simulink model "MODELO"  (R2024a)
settings: Solver=VariableStepAuto  StartTime=0.0  StopTime=10  RelTol=1e-3
libraries: simulink x2
settings Model: Creator=LENOVO  LastModifiedBy=LENOVO

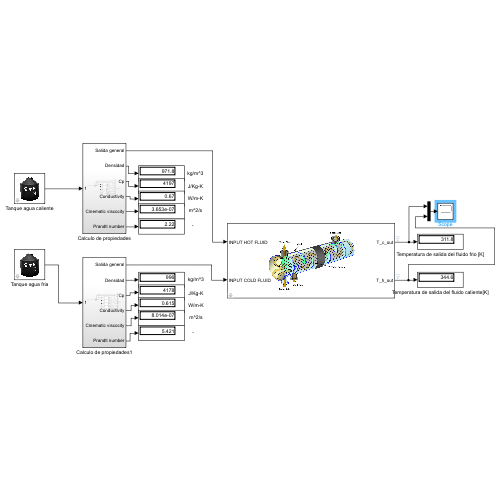
[thumbnail: Simulink's stored preview of the top-level diagram]
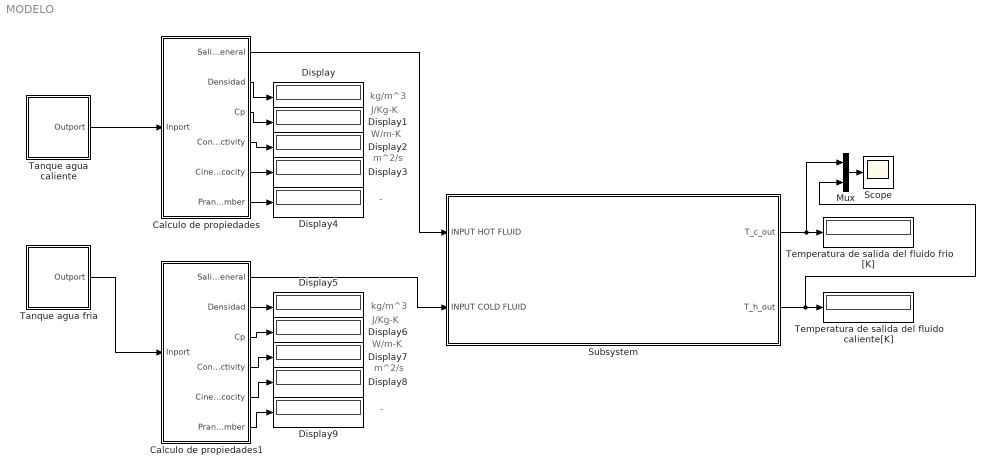
== system MODELO ==
  note: -
  note: m^2/s
  note: W/m-K
  note: J/Kg-K
  note: kg/m^3
  note: W/m-K
  note: -
  note: kg/m^3
  note: m^2/s
  note: J/Kg-K
  Calculo de propiedades : Subsystem
  Calculo de propiedades1 : Subsystem
  Display{,1..9} (10 alike) : Display
  Mux : Mux  Inputs=2
  Scope : Scope
  Subsystem : Subsystem  mask{jc=1.05, jl=1, jb=1, js=0.7065, jr=1, rfi=0, rfo=0}
      mask prompts: rfi "Factor de ensuciemiento dentro de los tubos"; rfo "Factor de ensuciemiento de la coraza"
      mask DialogControl Control2 Prompt: Introduzca los factores de corrección dados por el método de Bell-Delaware
      mask DialogControl Control3 Prompt: Introduzca los factores de ensuciamiento
      mask Display: image('HX.png', [0,0,0,0,90,90]);
  Tanque agua caliente : Subsystem  mask{Temp=80+273.15, ifCaudal=off, caudal=90, m_dot=10, area=2}
      mask prompts: Temp "Temperatura"; ifCaudal "Usar caudal"; m_dot "Flujo másico"
      mask Display: image('tanque_img.webp');
  Tanque agua fria : Subsystem  mask{Temp=30+273.15, ifCaudal=off, caudal=90, m_dot=3, area=2}
      mask prompts: Temp "Temperatura"; ifCaudal "Usar caudal"; m_dot "Flujo másico"
      mask Display: image('tanque_img.webp');
  Temperatura de salida del fluido caliente[K] : Display
  Temperatura de salida del fluido frio [K] : Display
  wires:
  Tanque agua caliente/1(Outport) -> Calculo de propiedades/1(Inport)
  Calculo de propiedades/2(Densidad) -> Display/1
  Calculo de propiedades/3(Cp) -> Display1/1
  Calculo de propiedades/4(Conductivity) -> Display2/1
  Calculo de propiedades/5(Cinematic viscocity) -> Display3/1
  Calculo de propiedades/6(Prandtl number) -> Display4/1
  Calculo de propiedades/1(Salida general) -> Subsystem/1(INPUT HOT FLUID)
  Tanque agua fria/1(Outport) -> Calculo de propiedades1/1(Inport)
  Calculo de propiedades1/2(Densidad) -> Display5/1
  Calculo de propiedades1/3(Cp) -> Display6/1
  Calculo de propiedades1/4(Conductivity) -> Display7/1
  Calculo de propiedades1/5(Cinematic viscocity) -> Display8/1
  Calculo de propiedades1/6(Prandtl number) -> Display9/1
  Calculo de propiedades1/1(Salida general) -> Subsystem/2(INPUT COLD FLUID)
  Subsystem/1(T_c_out) -> Mux/1, Temperatura de salida del fluido frio [K]/1
  Subsystem/2(T_h_out) -> Mux/2, Temperatura de salida del fluido caliente[K]/1
  Mux/1 -> Scope/1

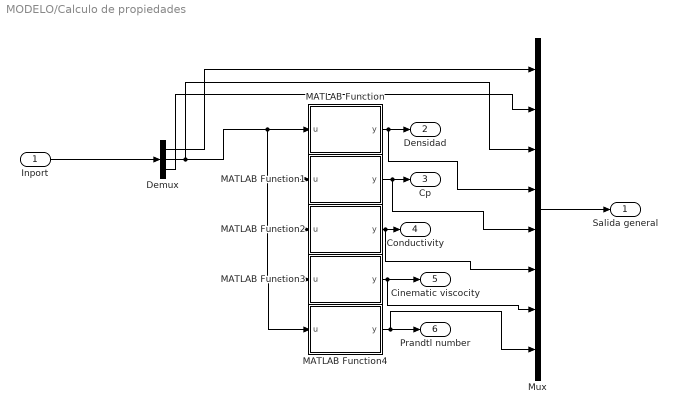
== system MODELO/Calculo de propiedades ==
  Inport : Inport
  Demux : Demux  Outputs=3
  MATLAB Function : MATLAB Function  TreatAsAtomicUnit=on
  MATLAB Function1 : MATLAB Function  TreatAsAtomicUnit=on
  MATLAB Function2 : MATLAB Function  TreatAsAtomicUnit=on
  MATLAB Function3 : MATLAB Function  TreatAsAtomicUnit=on
  MATLAB Function4 : MATLAB Function  TreatAsAtomicUnit=on
  Mux : Mux  Inputs=8
  Salida general : Outport
  Densidad : Outport  Port=2
  Cp : Outport  Port=3
  Conductivity : Outport  Port=4
  Cinematic viscocity : Outport  Port=5
  Prandtl number : Outport  Port=6
  wires:
  Inport/1 -> Demux/1
  Demux/1 -> Mux/1
  Demux/2 -> Mux/3, MATLAB Function4/1(u), MATLAB Function3/1(u), MATLAB Function2/1(u), MATLAB Function1/1(u), MATLAB Function/1(u)
  Demux/3 -> Mux/2
  MATLAB Function/1(y) -> Mux/4, Densidad/1
  MATLAB Function1/1(y) -> Mux/5, Cp/1
  MATLAB Function2/1(y) -> Mux/6, Conductivity/1
  MATLAB Function3/1(y) -> Mux/7, Cinematic viscocity/1
  MATLAB Function4/1(y) -> Mux/8, Prandtl number/1
  Mux/1 -> Salida general/1

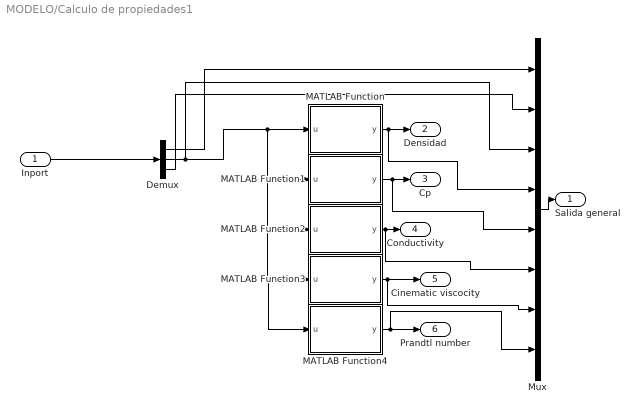
== system MODELO/Calculo de propiedades1 ==
  Inport : Inport
  Demux : Demux  Outputs=3
  MATLAB Function : MATLAB Function  TreatAsAtomicUnit=on
  MATLAB Function1 : MATLAB Function  TreatAsAtomicUnit=on
  MATLAB Function2 : MATLAB Function  TreatAsAtomicUnit=on
  MATLAB Function3 : MATLAB Function  TreatAsAtomicUnit=on
  MATLAB Function4 : MATLAB Function  TreatAsAtomicUnit=on
  Mux : Mux  Inputs=8
  Salida general : Outport
  Densidad : Outport  Port=2
  Cp : Outport  Port=3
  Conductivity : Outport  Port=4
  Cinematic viscocity : Outport  Port=5
  Prandtl number : Outport  Port=6
  wires:
  Inport/1 -> Demux/1
  Demux/1 -> Mux/1
  Demux/2 -> Mux/3, MATLAB Function4/1(u), MATLAB Function3/1(u), MATLAB Function2/1(u), MATLAB Function1/1(u), MATLAB Function/1(u)
  Demux/3 -> Mux/2
  MATLAB Function/1(y) -> Mux/4, Densidad/1
  MATLAB Function1/1(y) -> Mux/5, Cp/1
  MATLAB Function2/1(y) -> Mux/6, Conductivity/1
  MATLAB Function3/1(y) -> Mux/7, Cinematic viscocity/1
  MATLAB Function4/1(y) -> Mux/8, Prandtl number/1
  Mux/1 -> Salida general/1

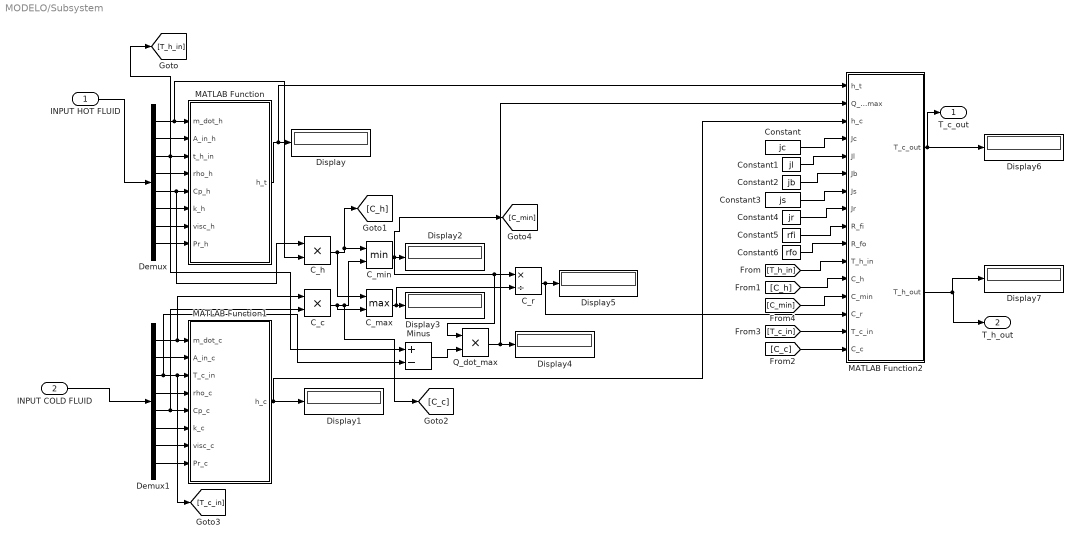
== system MODELO/Subsystem ==
  INPUT HOT FLUID : Inport
  INPUT COLD FLUID : Inport  Port=2
  C_c : Product
  C_h : Product
  C_max : MinMax  Function=max  Inputs=2
  C_min : MinMax  Inputs=2
  C_r : Product  Inputs=*/
  Constant : Constant  Value=jc
  Constant1 : Constant  Value=jl
  Constant2 : Constant  Value=jb
  Constant3 : Constant  Value=js
  Constant4 : Constant  Value=jr
  Constant5 : Constant  Value=rfi
  Constant6 : Constant  Value=rfo
  Demux : Demux  Outputs=8
  Demux1 : Demux  Outputs=8
  Display{,1..7} (8 alike) : Display
  MATLAB Function : MATLAB Function  TreatAsAtomicUnit=on
  MATLAB Function1 : MATLAB Function  TreatAsAtomicUnit=on
  MATLAB Function2 : MATLAB Function  TreatAsAtomicUnit=on
  Minus : Sum  Inputs=+-
  Q_dot_max : Product
  T_c_out : Outport
  T_h_out : Outport  Port=2
  wires:
  INPUT HOT FLUID/1 -> Demux/1
  Demux/1 -> C_h/2, MATLAB Function/1(m_dot_h)
  Demux/2 -> MATLAB Function/2(A_in_h)
  Demux/3 -> [T_h_in], Minus/1, MATLAB Function/3(t_h_in)
  Demux/4 -> MATLAB Function/4(rho_h)
  Demux/7 -> MATLAB Function/7(visc_h)
  Demux/8 -> MATLAB Function/8(Pr_h)
  Demux1/1 -> C_c/1, MATLAB Function1/1(m_dot_c)
  Demux1/2 -> MATLAB Function1/2(A_in_c)
  Demux1/3 -> Minus/2, [T_c_in], MATLAB Function1/3(T_c_in)
  Demux1/4 -> MATLAB Function1/4(rho_c)
  Demux1/5 -> C_c/2, MATLAB Function1/5(Cp_c)
  Demux1/6 -> MATLAB Function1/6(k_c)
  Demux1/7 -> MATLAB Function1/7(visc_c)
  Demux1/8 -> MATLAB Function1/8(Pr_c)
  INPUT COLD FLUID/1 -> Demux1/1
  MATLAB Function/1(h_t) -> MATLAB Function2/1(h_t), Display/1
  MATLAB Function1/1(h_c) -> MATLAB Function2/3(h_c), Display1/1
  Demux/5 -> C_h/1, MATLAB Function/5(Cp_h)
  Demux/6 -> MATLAB Function/6(k_h)
  C_h/1 -> C_max/1, [C_h], C_min/1
  C_c/1 -> C_max/2, [C_c], C_min/2
  C_max/1 -> C_r/2, Display3/1
  C_min/1 -> [C_min], Q_dot_max/1, C_r/1, Display2/1
  Minus/1 -> Q_dot_max/2
  Q_dot_max/1 -> MATLAB Function2/2(Q_dot_max), Display4/1
  C_r/1 -> MATLAB Function2/14(C_r), Display5/1
  Constant/1 -> MATLAB Function2/4(Jc)
  Constant2/1 -> MATLAB Function2/6(Jb)
  Constant1/1 -> MATLAB Function2/5(Jl)
  Constant3/1 -> MATLAB Function2/7(Js)
  Constant4/1 -> MATLAB Function2/8(Jr)
  Constant5/1 -> MATLAB Function2/9(R_fi)
  Constant6/1 -> MATLAB Function2/10(R_fo)
  [T_h_in] -> MATLAB Function2/11(T_h_in)
  [C_h] -> MATLAB Function2/12(C_h)
  [C_c] -> MATLAB Function2/16(C_c)
  [T_c_in] -> MATLAB Function2/15(T_c_in)
  [C_min] -> MATLAB Function2/13(C_min)
  MATLAB Function2/1(T_c_out) -> T_c_out/1, Display6/1
  MATLAB Function2/2(T_h_out) -> Display7/1, T_h_out/1

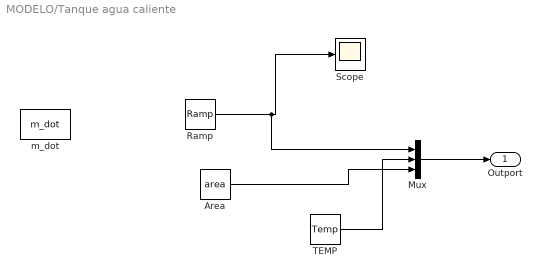
== system MODELO/Tanque agua caliente ==
  Area : Constant  Value=area
  Mux : Mux  Inputs=3
  Ramp : simulink/Sources/Ramp  slope=1  start=0  InitialOutput=0
  Scope : Scope
  TEMP : Constant  Value=Temp
  m_dot : Constant  Value=m_dot
  Outport : Outport
  wires:
  TEMP/1 -> Mux/2
  Area/1 -> Mux/3
  Mux/1 -> Outport/1
  Ramp/1 -> Mux/1, Scope/1

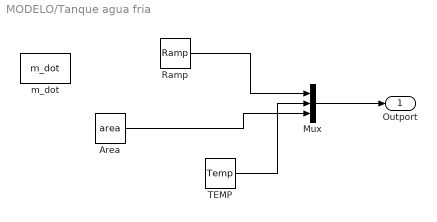
== system MODELO/Tanque agua fria ==
  Area : Constant  Value=area
  Mux : Mux  Inputs=3
  Ramp : simulink/Sources/Ramp  slope=1  start=0  InitialOutput=0
  TEMP : Constant  Value=Temp
  m_dot : Constant  Value=m_dot
  Outport : Outport
  wires:
  TEMP/1 -> Mux/2
  Area/1 -> Mux/3
  Mux/1 -> Outport/1
  Ramp/1 -> Mux/1

== matlab function MODELO/Calculo de propiedades1/MATLAB Function2 ==
  data: u input; y output
function y = fcn(u)
    temp_vector=273.16:5:373.16;
    k_vector = [0.56 0.571 0.580 0.589 0.598 0.607 0.615 0.623 0.631 0.637 ...
            0.644 0.649 0.654 0.659 0.663 0.667 0.670 0.673 0.675 0.677 ...
            0.679];
    fluid_k = interp1(temp_vector, k_vector, u);

y = fluid_k;

== matlab function MODELO/Calculo de propiedades1/MATLAB Function3 ==
  data: u input; y output
function y = fcn(u)
    temp_vector=273.16:5:373.16;
    density_vector=[999.8 999.9 999.7 999.1 998.0 997.0 996.0 994.0 992.1 990.1 988.1 985.2 983.3 980.4 977.5 974.7 971.8 968.1 965.3 961.5 957.9];
    mu_vector = [1.792e-3 1.519e-3 1.307e-3 1.138e-3 1.002e-3 ...
             0.891e-3 0.798e-3 0.720e-3 0.653e-3 0.596e-3 ...
             0.547e-3 0.467e-3 0.467e-3 0.433e-3 0.404e-3 ...
             0.378e-3 0.355e-3 0.333e-3 0.315e-3 0.297e-3 ...
             0.282e-3];
    v_vector=mu_vector./density_vector;
    
    fluid_v = interp1(temp_vector, v_vector, u);

y = fluid_v;

== matlab function MODELO/Calculo de propiedades1/MATLAB Function4 ==
  data: u input; y output
function y = fcn(u)
    temp_vector=273.16:5:373.16;
    pr_vector = [13.5 11.2 9.45 8.09 7.01 6.14 5.42 4.83 ...
             4.32 3.91 3.55 3.25 2.99 2.75 2.55 2.38 ...
             2.22 2.08 1.96 1.85 1.75];
    fluid_pr = interp1(temp_vector, pr_vector, u);

y = fluid_pr;

== matlab function MODELO/Subsystem/MATLAB Function2 ==
  data: h_t input; Q_dot_max input; T_c_out output; h_c input; T_h_out output; Jc input; Jl input; Jb input; Js input; Jr input; R_fi input; R_fo input; T_h_in input; C_h input; C_min input; C_r input; T_c_in input; C_c input
function [T_c_out, T_h_out] = fcn(h_t, Q_dot_max, h_c, Jc, Jl, Jb, Js, Jr, R_fi, R_fo, T_h_in, C_h, C_min, C_r, T_c_in, C_c)
    d_t=0.0072;
    L_t=0.506;
    d_t_in=0.006;
    N_t=167;
    % Corregir el coeficiente de transferencia de calor h_c
    h_c_corregido = h_c * Jc * Jl * Jb * Js * Jr;

    % Parámetros del intercambiador de calor
    k_tubos = 121.42; % Conductividad térmica de los tubos [W/m·K]

    % Calcular las áreas de superficie
    A_s = pi * d_t * L_t * N_t; % Área superficial del lado caliente (exterior de los tubos)
    A_o = pi * d_t * L_t * N_t; % Área superficial del lado frío (exterior de los tubos)
    A_i = pi * d_t_in * L_t * N_t; % Área superficial del lado interior de los tubos

    % Calcular la resistencia total
    R_total = (1 / (h_c_corregido * A_o)) + (1 / (h_t * A_i)) + R_fo / A_o + R_fi / A_i;

    % Calcular el coeficiente global de transferencia de calor U
    U = 1 / (R_total*A_s);

    % Calcular el número de unidades de transferencia (NTU)
    NTU = (U * A_s) / C_min;

    % Calcular la efectividad del intercambiador de calor usando la fórmula para un intercambiador de flujo cruzado con un número infinito de placas
    epsilon=2*(1+C_r+sqrt(1+C_r^2)*((1+exp(-NTU*sqrt(1+C_r^2)))/(1-exp(-NTU*sqrt(1+C_r^2)))))^-1;
    epsilon2=(1-exp(-NTU*(1+C_r)))/(1+C_r);


    % Calcular la tasa de transferencia de calor real
    Q_dot = epsilon * Q_dot_max;

    % Calcular las temperaturas de salida
    T_h_out = T_h_in - Q_dot / C_h;
    T_c_out = T_c_in + Q_dot / C_c;

end

== matlab function MODELO/Calculo de propiedades/MATLAB Function1 ==
  data: u input; y output
function y = fcn(u)
    temp_vector=273.16:5:373.16;
    cp_vector=[4217 4205 4194 4186 4182 4180 4178 4178 4179 4180 4181 4183 4185 4187 4190 4193 4197 4201 4206 4212 4217];
    fluid_cp = interp1(temp_vector, cp_vector, u);

y = fluid_cp;

== matlab function MODELO/Calculo de propiedades/MATLAB Function ==
  data: u input; y output
function y = fcn(u)
    temp_vector=273.16:5:373.16;
    density_vector=[999.8 999.9 999.7 999.1 998.0 997.0 996.0 994.0 992.1 990.1 988.1 985.2 983.3 980.4 977.5 974.7 971.8 968.1 965.3 961.5 957.9];
    fluid_density = interp1(temp_vector, density_vector, u);

y = fluid_density;

== matlab function MODELO/Calculo de propiedades/MATLAB Function2 ==
  data: u input; y output
function y = fcn(u)
    temp_vector=273.16:5:373.16;
    k_vector = [0.56 0.571 0.580 0.589 0.598 0.607 0.615 0.623 0.631 0.637 ...
            0.644 0.649 0.654 0.659 0.663 0.667 0.670 0.673 0.675 0.677 ...
            0.679];
    fluid_k = interp1(temp_vector, k_vector, u);

y = fluid_k;

== matlab function MODELO/Calculo de propiedades/MATLAB Function3 ==
  data: u input; y output
function y = fcn(u)
    temp_vector=273.16:5:373.16;
    density_vector=[999.8 999.9 999.7 999.1 998.0 997.0 996.0 994.0 992.1 990.1 988.1 985.2 983.3 980.4 977.5 974.7 971.8 968.1 965.3 961.5 957.9];
    mu_vector = [1.792e-3 1.519e-3 1.307e-3 1.138e-3 1.002e-3 ...
             0.891e-3 0.798e-3 0.720e-3 0.653e-3 0.596e-3 ...
             0.547e-3 0.467e-3 0.467e-3 0.433e-3 0.404e-3 ...
             0.378e-3 0.355e-3 0.333e-3 0.315e-3 0.297e-3 ...
             0.282e-3];
    v_vector=mu_vector./density_vector;
    
    fluid_v = interp1(temp_vector, v_vector, u);

y = fluid_v;

== matlab function MODELO/Calculo de propiedades/MATLAB Function4 ==
  data: u input; y output
function y = fcn(u)
    temp_vector=273.16:5:373.16;
    pr_vector = [13.5 11.2 9.45 8.09 7.01 6.14 5.42 4.83 ...
             4.32 3.91 3.55 3.25 2.99 2.75 2.55 2.38 ...
             2.22 2.08 1.96 1.85 1.75];
    fluid_pr = interp1(temp_vector, pr_vector, u);

y = fluid_pr;

== matlab function MODELO/Subsystem/MATLAB Function ==
  data: m_dot_h input; h_t output; A_in_h input; t_h_in input; rho_h input; Cp_h input; k_h input; visc_h input; Pr_h input
function h_t = fcn(m_dot_h, A_in_h, t_h_in, rho_h, Cp_h, k_h, visc_h, Pr_h)

    % Parámetros fijos o constantes (pueden ser pasados como argumentos si varían)
    d_t = 0.0072; % Diámetro del tubo [m]
    d_t_in = 0.006; % Diámetro interno del tubo [m]
    L_t = 0.506; % Longitud del tubo [m]
    D_entrada_hot = 0.079; % Diámetro de entrada del fluido caliente [m]

    % Área de la entrada del fluido caliente
    A_h = (pi / 4) * D_entrada_hot^2;

    % Velocidad del fluido caliente
    vel_h = m_dot_h / (rho_h * A_h);

    % Número de Reynolds del fluido caliente
    Re_h = (D_entrada_hot * vel_h) / visc_h;

    % Número de Nusselt del fluido caliente
    if Re_h < 2100
        % Flujo laminar
        Nu_h = 1.86 * (Re_h * Pr_h * (d_t / L_t))^0.5 * Pr_h^(1/3);
    elseif Re_h >= 2100 && Re_h <= 10000
        % Flujo de transición
        Nu_h = 0.116 * (Re_h^(2/3) - 125) * (1 + (d_t / L_t)^(2/3) * Pr_h^(1/3));
    else
        % Flujo turbulento
        Nu_h = 0.023 * Re_h^0.8 * Pr_h^0.4;
    end

    % Coeficiente de transferencia de calor por convección
    h_t = (k_h * Nu_h) / D_entrada_hot;

end

== matlab function MODELO/Subsystem/MATLAB Function1 ==
  data: m_dot_c input; h_c output; A_in_c input; T_c_in input; rho_c input; Cp_c input; k_c input; visc_c input; Pr_c input
function h_c = fcn(m_dot_c, A_in_c, T_c_in, rho_c, Cp_c, k_c, visc_c, Pr_c)

    % Parámetros fijos o constantes (pueden ser pasados como argumentos si varían)
    D_c = 0.506; % Diámetro de la coraza [m]
    L_c = 0.506; % Longitud de la coraza [m]
    D_entrada_cold = 0.044; % Diámetro de entrada del fluido frío [m]
    D_eq_c = 0.113; % Diámetro equivalente [m]

    % Área de la entrada del fluido frío
    A_c = (pi / 4) * D_entrada_cold^2;

    % Velocidad del fluido frío
    vel_c = m_dot_c / (rho_c * A_c);

    % Número de Reynolds del fluido frío
    Re_c = (D_entrada_cold * vel_c) / visc_c;

    % Número de Nusselt del fluido frío
    if Re_c < 2100
        % Flujo laminar
        Nu_c = 1.86 * (Re_c * Pr_c * D_c / L_c)^0.5 * Pr_c^(1/3);
    elseif Re_c >= 2100 && Re_c <= 10000
        % Flujo de transición
        Nu_c = 0.116 * (Re_c^(2/3) - 125) * (1 + (D_eq_c / L_c)^(2/3) * Pr_c^(1/3));
    else
        % Flujo turbulento
        Nu_c = 0.023 * Re_c^0.8 * Pr_c^(1/3);
    end

    % Coeficiente de transferencia de calor por convección
    h_c = (k_c * Nu_c) / D_entrada_cold;

end

== matlab function MODELO/Calculo de propiedades1/MATLAB Function ==
  data: u input; y output
function y = fcn(u)
    temp_vector=273.16:5:373.16;
    density_vector=[999.8 999.9 999.7 999.1 998.0 997.0 996.0 994.0 992.1 990.1 988.1 985.2 983.3 980.4 977.5 974.7 971.8 968.1 965.3 961.5 957.9];
    fluid_density = interp1(temp_vector, density_vector, u);

y = fluid_density;

== matlab function MODELO/Calculo de propiedades1/MATLAB Function1 ==
  data: u input; y output
function y = fcn(u)
    temp_vector=273.16:5:373.16;
    cp_vector=[4217 4205 4194 4186 4182 4180 4178 4178 4179 4180 4181 4183 4185 4187 4190 4193 4197 4201 4206 4212 4217];
    fluid_cp = interp1(temp_vector, cp_vector, u);

y = fluid_cp;
